simulink model "MEEN432_Project1_Part2_Op1"  (R2023b)
settings: Solver=ode45  StartTime=0.0  StopTime=10  FixedStep=0.1  RelTol=1e-3
values from neighbouring files (symbols this model uses):
  b1 = 1    [MEEN432_Project1_Part2.m]
  b2 = 1    [MEEN432_Project1_Part2.m]
  const_torque = 1    [MEEN432_Project1_Part2.m]    (also in Project1_Part1.m = 0)
  J1 = 100    [MEEN432_Project1_Part2.m]
  J2 = 1    [MEEN432_Project1_Part2.m]
  k = k_int(i)    [MEEN432_Project1_Part2.m]
  omega0 = 0    [MEEN432_Project1_Part2.m]    (also in Project1_Part1.m = omega0_values(l))
  theta0 = 0    [MEEN432_Project1_Part2.m]    (also in Project1_Part1.m)
settings Model: Creator=sgopalswamy  LastModifiedBy=flare
settings SolverCC: AlgebraicLoopSolver=TrustRegion
settings DataIOCC: ReturnWorkspaceOutputsName=out1
settings DebuggingCC: UnconnectedInputMsg=warning  UnconnectedOutputMsg=warning  UnconnectedLineMsg=warning  ArithmeticOperatorsInVariantConditions=warning
settings ModelReferenceCC: EnableRefExpFcnMdlSchedulingChecks=on
settings SFSimCC: SimUseLocalCustomCode=off  CustomCodeUndefinedFunction=UseInterfaceOnly
settings RTWCC: RTWUseLocalCustomCode=off
settings CodeAppCC: StateflowObjectComments=on

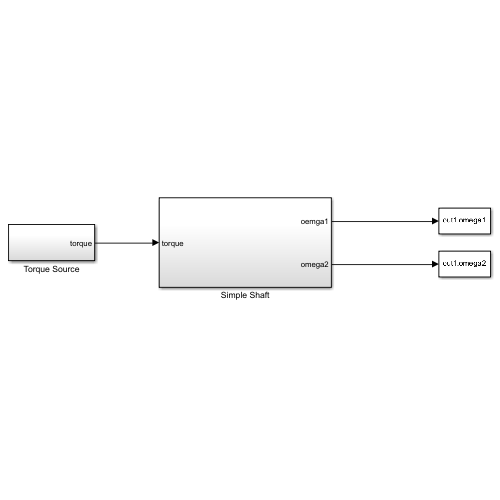
[thumbnail: Simulink's stored preview of the top-level diagram]
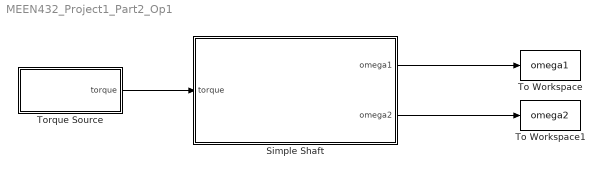
== system MEEN432_Project1_Part2_Op1 ==
  Simple Shaft : Subsystem
  To Workspace : ToWorkspace  VariableName=omega1  SaveFormat=Timeseries  SampleTime=-1
  To Workspace1 : ToWorkspace  VariableName=omega2  SaveFormat=Timeseries  SampleTime=-1
  Torque Source : Subsystem
  wires:
  Torque Source/1(torque) -> Simple Shaft/1(torque)
  Simple Shaft/1(omega1) -> To Workspace/1
  Simple Shaft/2(omega2) -> To Workspace1/1

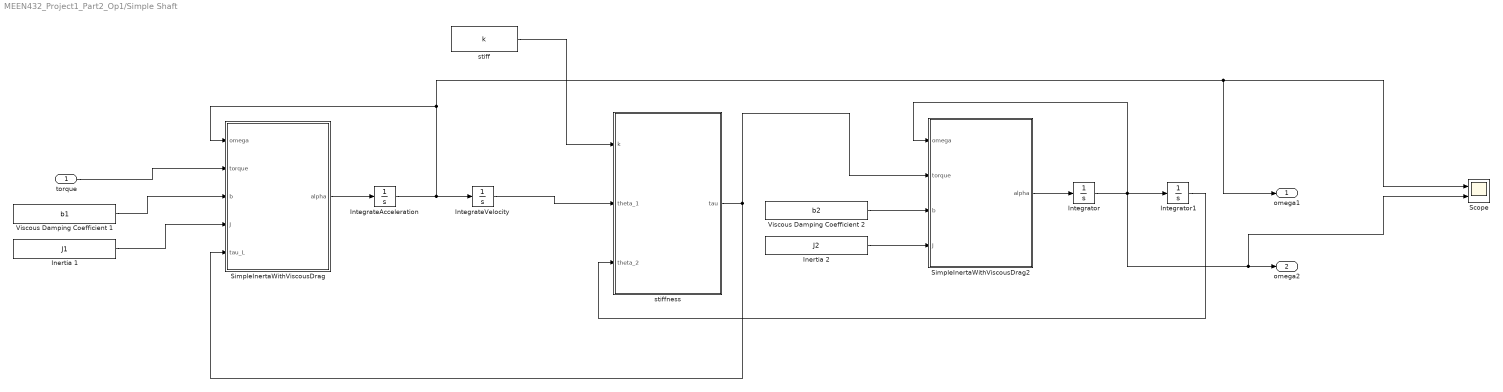
== system MEEN432_Project1_Part2_Op1/Simple Shaft ==
  torque : Inport
  Inertia 1 : Constant  Value=J1
  Inertia 2 : Constant  Value=J2
  IntegrateAcceleration : Integrator  InitialCondition=omega0
  IntegrateVelocity : Integrator  InitialCondition=theta0
  Integrator : Integrator
  Integrator1 : Integrator
  Scope : Scope  NumInputPorts=2
  SimpleInertaWithViscousDrag : MATLAB Function  TreatAsAtomicUnit=on
  SimpleInertaWithViscousDrag2 : MATLAB Function  TreatAsAtomicUnit=on
  Viscous Damping Coefficient 1 : Constant  Value=b1
  Viscous Damping Coefficient 2 : Constant  Value=b2
  stiff : Constant  Value=k
  stiffness : MATLAB Function  TreatAsAtomicUnit=on
  omega1 : Outport
  omega2 : Outport  Port=2
  wires:
  IntegrateAcceleration/1 -> SimpleInertaWithViscousDrag/1(omega), omega1/1, Scope/1, IntegrateVelocity/1
  IntegrateVelocity/1 -> stiffness/2(theta_1)
  SimpleInertaWithViscousDrag/1(alpha) -> IntegrateAcceleration/1
  torque/1 -> SimpleInertaWithViscousDrag/2(torque)
  Viscous Damping Coefficient 1/1 -> SimpleInertaWithViscousDrag/3(b)
  Inertia 1/1 -> SimpleInertaWithViscousDrag/4(J)
  stiff/1 -> stiffness/1(k)
  SimpleInertaWithViscousDrag2/1(alpha) -> Integrator/1
  Integrator/1 -> Scope/2, omega2/1, SimpleInertaWithViscousDrag2/1(omega), Integrator1/1
  Integrator1/1 -> stiffness/3(theta_2)
  stiffness/1(tau) -> SimpleInertaWithViscousDrag2/2(torque), SimpleInertaWithViscousDrag/5(tau_L)
  Viscous Damping Coefficient 2/1 -> SimpleInertaWithViscousDrag2/3(b)
  Inertia 2/1 -> SimpleInertaWithViscousDrag2/4(J)

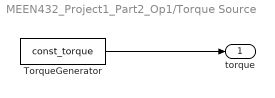
== system MEEN432_Project1_Part2_Op1/Torque Source ==
  TorqueGenerator : Constant  Value=const_torque
  torque : Outport
  wires:
  TorqueGenerator/1 -> torque/1

== matlab function MEEN432_Project1_Part2_Op1/Simple Shaft/stiffness ==
  data: k input; tau output; theta_1 input; theta_2 input
function tau = fcn(k, theta_1, theta_2)

tau = k*(theta_1 - theta_2);

== matlab function MEEN432_Project1_Part2_Op1/Simple Shaft/SimpleInertaWithViscousDrag ==
  data: omega input; torque input; alpha output; b input; J input; tau_L input
function alpha = fcn(omega, torque,b, J, tau_L)
alpha = (torque - tau_L - omega * b)/J;

== matlab function MEEN432_Project1_Part2_Op1/Simple Shaft/SimpleInertaWithViscousDrag2 ==
  data: omega input; torque input; alpha output; b input; J input
function alpha = fcn(omega, torque,b, J)
alpha = (torque - omega * b)/J;
